simulink model "FirstOrderSystemAdjustment"  (R2013b)
settings: Solver=ode45  StartTime=0.0  StopTime=15  RelTol=1e-3
settings Model: Creator=MMSA  LastModifiedBy=MMSA
settings SolverCC: ZeroCrossAlgorithm=Adaptive  PositivePriorityOrder=on
settings HardwareCC: ProdBitPerPointer=64  ProdHWDeviceType=Generic->64-bit Embedded Processor (LLP64)

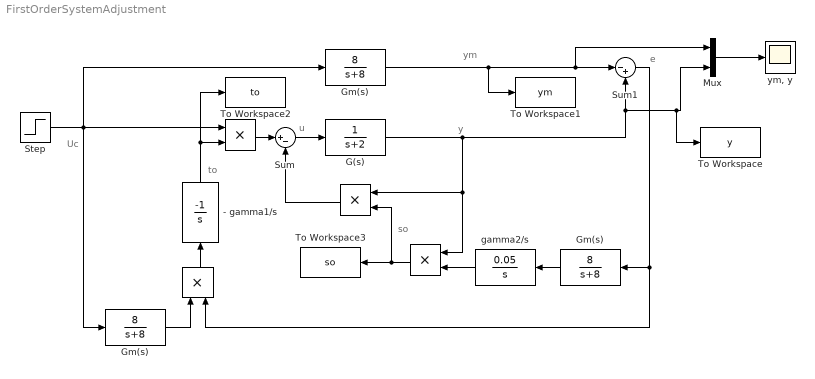
== system FirstOrderSystemAdjustment ==
  note: so
  note: to
  note: Uc
  note: u
  note: e
  note: y
  note: ym
  " " : Product
  "  " : Product
  " " : Product
  "   " : Product
  - gamma1/s : TransferFcn  Numerator=[-1]  Denominator=[1 0]
  G(s) : TransferFcn  Denominator=[1 2]
  Gm(s) : TransferFcn  Numerator=[8]  Denominator=[1 8]
  "Gm(s)  " : TransferFcn  Numerator=[8]  Denominator=[1 8]
  "Gm(s)   " : TransferFcn  Numerator=[8]  Denominator=[1 8]
  Mux : Mux  Inputs=2
  Step : Step  Time=0  SampleTime=0
  Sum : Sum  Inputs=|+-
  Sum1 : Sum  Inputs=|-+
  To Workspace : ToWorkspace  VariableName=y  SampleTime=-1
  To Workspace1 : ToWorkspace  VariableName=ym  SampleTime=-1
  To Workspace2 : ToWorkspace  VariableName=to  SampleTime=-1
  To Workspace3 : ToWorkspace  VariableName=so  SampleTime=-1
  gamma2/s : TransferFcn  Numerator=[0.05]  Denominator=[1 0]
  "ym, y " : Scope
  wires:
  Sum/1 -> G(s)/1
  Step/1 -> "   "/1, "Gm(s)  "/1, Gm(s)/1
  Gm(s)/1 -> To Workspace1/1, Mux/1, Sum1/1
  G(s)/1 -> To Workspace/1, Mux/2, Sum1/2, " "/1, "  "/1
  Mux/1 -> "ym, y "/1
  "   "/1 -> Sum/1
  "Gm(s)  "/1 -> " "/1
  Sum1/1 -> " "/2, "Gm(s)   "/1
  " "/1 -> - gamma1/s/1
  - gamma1/s/1 -> To Workspace2/1, "   "/2
  "  "/1 -> Sum/2
  "Gm(s)   "/1 -> gamma2/s/1
  gamma2/s/1 -> " "/2
  " "/1 -> "  "/2, To Workspace3/1
